simulink model "Modelo_Tanque"  (R2022a)
settings: Solver=FixedStepAuto  StartTime=0.0  StopTime=18600  FixedStep=1e-3  RelTol=1e-3
libraries: simulink x2
settings Model: Creator=User  LastModifiedBy=User
settings DebuggingCC: UnconnectedInputMsg=warning  UnconnectedOutputMsg=warning  UnconnectedLineMsg=warning
settings RTWCC: DLArmComputeVersion=19.05

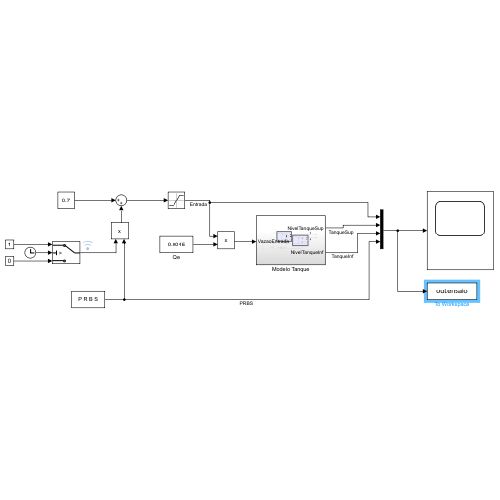
[thumbnail: Simulink's stored preview of the top-level diagram]
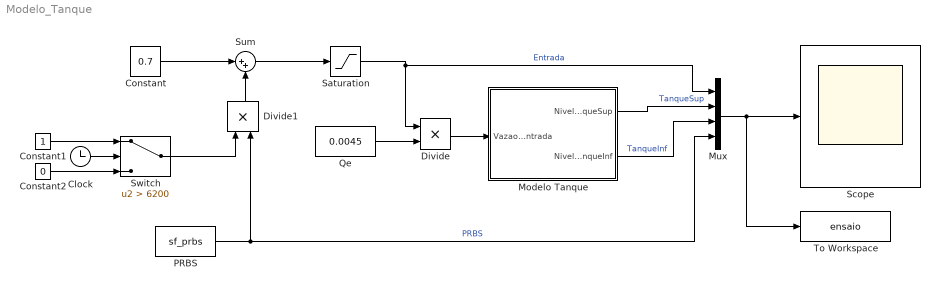
== system Modelo_Tanque ==
  Clock : Clock
  Constant : Constant  Value=0.7
  Constant1 : Constant
  Constant2 : Constant  Value=0
  Divide : Product  Inputs=**
  Divide1 : Product  Inputs=**
  Modelo Tanque : Subsystem
  Mux : Mux
  PRBS : S-Function  FunctionName=sf_prbs  Parameters=K,N,Ts  SFunctionDeploymentMode=off  EnableBusSupport=off  mask{K=0.15, N=5, Ts=200}
      mask prompts: K "Ganho (K):"; N "Número de Células (usar 5, 7 ou 10):"; Ts "Tb (seg):"
      mask Display: disp('P R B S')
  Qe : Constant  Value=0.0045
  Saturation : Saturate  UpperLimit=1  LowerLimit=0
  Scope : Scope
  Sum : Sum  Inputs=|++
  Switch : Switch  Criteria=u2 > Threshold  Threshold=6200  SaturateOnIntegerOverflow=off  InputSameDT=off
  To Workspace : ToWorkspace  VariableName=ensaio  SaveFormat=Timeseries  SampleTime=40
  wires:
  Qe/1 -> Divide/2
  Divide/1 -> Modelo Tanque/1(VazaoEntrada)
  Saturation/1 -> Divide/1, Mux/1  "Entrada"
  Sum/1 -> Saturation/1
  Modelo Tanque/1(NivelTanqueSup) -> Mux/2  "TanqueSup"
  Modelo Tanque/2(NivelTanqueInf) -> Mux/3  "TanqueInf"
  Constant/1 -> Sum/1
  Clock/1 -> Switch/2
  Constant1/1 -> Switch/1
  Constant2/1 -> Switch/3
  Switch/1 -> Divide1/1
  PRBS/1 -> Mux/4, Divide1/2  "PRBS"
  Divide1/1 -> Sum/2
  Mux/1 -> To Workspace/1, Scope/1

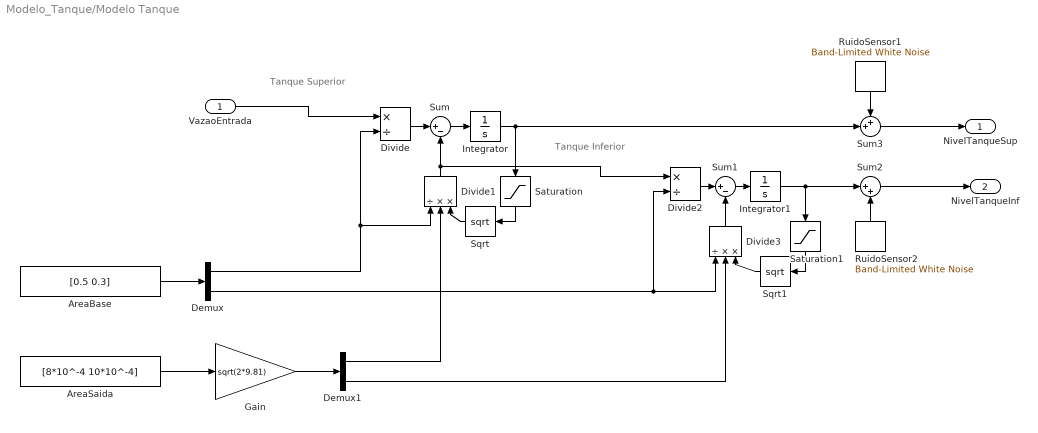
== system Modelo_Tanque/Modelo Tanque ==
  note: Tanque Inferior
  note: Tanque Superior
  VazaoEntrada : Inport
  AreaBase : Constant  Value=[0.5 0.3]
  AreaSaida : Constant  Value=[8*10^-4 10*10^-4]
  Demux : Demux  Outputs=2
  Demux1 : Demux  Outputs=2
  Divide : Product  Inputs=*/
  Divide1 : Product  Inputs=/**
  Divide2 : Product  Inputs=*/
  Divide3 : Product  Inputs=/**
  Gain : Gain  Gain=sqrt(2*9.81)
  Integrator : Integrator
  Integrator1 : Integrator
  RuidoSensor1 : simulink/Sources/Band-Limited White Noise  Cov=[0.00001]  Ts=1  seed=[23341]
  RuidoSensor2 : simulink/Sources/Band-Limited White Noise  Cov=[0.00001]  Ts=1  seed=[23341]
  Saturation : Saturate  UpperLimit=inf  LowerLimit=0
  Saturation1 : Saturate  UpperLimit=inf  LowerLimit=0
  Sqrt : Sqrt
  Sqrt1 : Sqrt
  Sum : Sum  Inputs=|+-
  Sum1 : Sum  Inputs=|+-
  Sum2 : Sum  Inputs=|++
  Sum3 : Sum  Inputs=++|
  NivelTanqueSup : Outport
  NivelTanqueInf : Outport  Port=2
  wires:
  AreaSaida/1 -> Gain/1
  AreaBase/1 -> Demux/1
  Gain/1 -> Demux1/1
  Sum3/1 -> NivelTanqueSup/1
  Integrator/1 -> Saturation/1, Sum3/2
  Demux/1 -> Divide/2, Divide1/1
  Divide/1 -> Sum/1
  Sum/1 -> Integrator/1
  Demux1/1 -> Divide1/2
  Sqrt/1 -> Divide1/3
  Integrator1/1 -> Sum2/1, Saturation1/1
  Demux1/2 -> Divide3/2
  Sqrt1/1 -> Divide3/3
  Divide3/1 -> Sum1/2
  Demux/2 -> Divide3/1, Divide2/2
  Sum1/1 -> Integrator1/1
  Divide2/1 -> Sum1/1
  Sum2/1 -> NivelTanqueInf/1
  RuidoSensor2/1 -> Sum2/2
  RuidoSensor1/1 -> Sum3/1
  VazaoEntrada/1 -> Divide/1
  Divide1/1 -> Divide2/1, Sum/2
  Saturation/1 -> Sqrt/1
  Saturation1/1 -> Sqrt1/1
